simulink model "extend_kalman"  (R2023b)
settings: Solver=FixedStepDiscrete  StartTime=0.0  StopTime=10000  RelTol=1e-3
undefined symbols (not defined in the file or in its folder): BMS_State_Enum, delta_t, dOCV, eta, M, M0, OCV_values, Q, R, R0, sigmaV, sigmaW, soc_values, taw, vbar
libraries: simulink x1
settings Model: DataDictionary=DD_EKF.sldd  Creator=Alkhouly  LastModifiedBy=user
settings OptimizationCC: DefaultParameterBehavior=Inlined  PassReuseOutputArgsAs=Individual arguments  ZeroExternalMemoryAtStartup=off  ZeroInternalMemoryAtStartup=off  OptimizeBlockOrder=speed  DifferentSizesBufferReuse=on  EfficientTunableParamExpr=on
settings DebuggingCC: ParameterTunabilityLossMsg=error  UnconnectedInputMsg=warning  UnconnectedOutputMsg=warning  UnconnectedLineMsg=warning
settings ModelReferenceCC: EnableRefExpFcnMdlSchedulingChecks=on
settings SFSimCC: MATLABDynamicMemAlloc=off
settings RTWCC: Description=Embedded Coder  SystemTargetFile=ert.tlc  GenCodeOnly=on  TemplateMakefile=ert_default_tmf  GenerateReport=on  Toolchain=Texas Instruments Code Composer Studio (C2000)  GenerateWebview=on  GenerateCodeMetricsReport=on  DLArmComputeVersion=19.05
settings CodeAppCC: ForceParamTrailComments=on  IgnoreCustomStorageClasses=off  MaxIdLength=51  OperatorAnnotations=on  SimulinkDataObjDesc=on  SFDataObjDesc=on  MangleLength=4  InsertBlockDesc=on
settings ERTTargetCC: UtilityFuncGeneration=Shared location  SuppressErrorStatus=on  SupportNonFinite=off  SupportComplex=off  ParenthesesLevel=Maximum  CastingMode=Standards  InlinedParameterPlacement=NonHierarchical  ERTCustomFileTemplate=example_file_process.tlc  PreserveExpressionOrder=on  PreserveIfCondition=on  EnableSignedLeftShifts=off  EnableSignedRightShifts=off

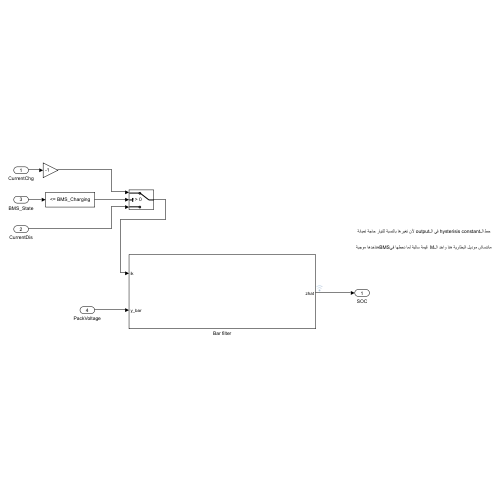
[thumbnail: Simulink's stored preview of the top-level diagram]
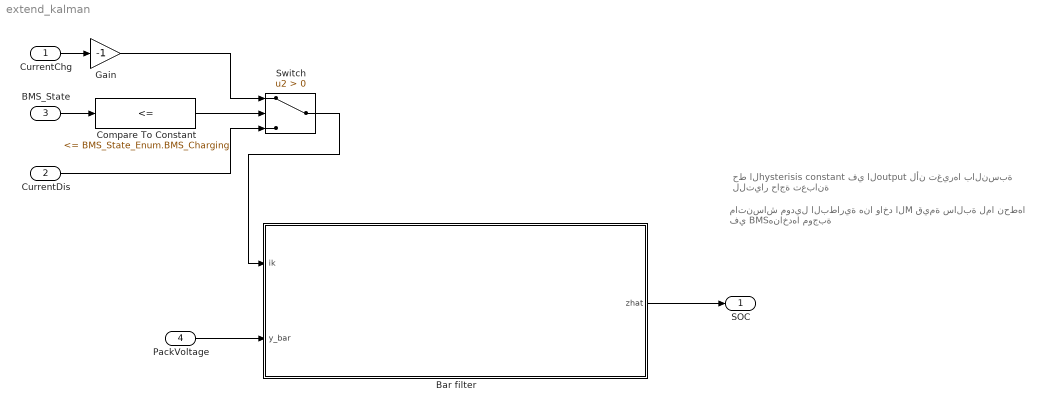
== system extend_kalman ==
  note: ماتنساش موديل البطارية هنا واخد الM قيمة سالبة لما نحطها في BMSهناخدها موجبة
  note: حط الhysterisis constant في الoutput لأن تغيرها بالنسبة للتيار حاجة تعبانة
  CurrentChg : Inport
  CurrentDis : Inport  Port=2
  BMS_State : Inport  Port=3
  PackVoltage : Inport  Port=4
  Bar filter : Subsystem
  Compare To Constant : simulink/Logic and Bit Operations/Compare To Constant  relop=<=  const=BMS_State_Enum.BMS_Charging  OutDataTypeStr=boolean
  Gain : Gain  Gain=-1
  Switch : Switch  Criteria=u2 > Threshold  SaturateOnIntegerOverflow=off  InputSameDT=off
  SOC : Outport
  wires:
  Bar filter/1(zhat) -> SOC/1
  PackVoltage/1 -> Bar filter/2(y_bar)
  CurrentChg/1 -> Gain/1
  CurrentDis/1 -> Switch/3
  Compare To Constant/1 -> Switch/2
  Gain/1 -> Switch/1
  BMS_State/1 -> Compare To Constant/1
  Switch/1 -> Bar filter/1(ik)

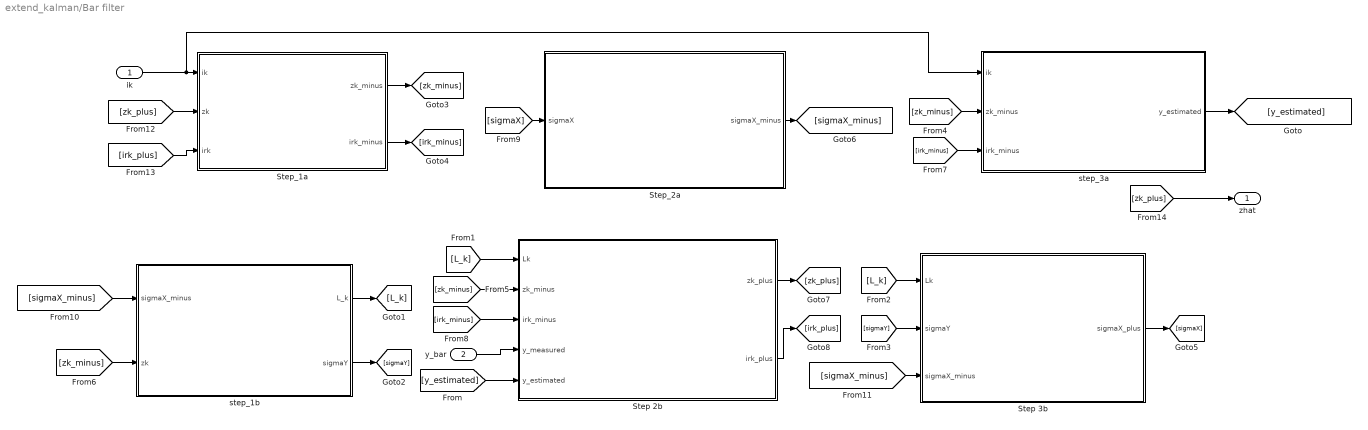
== system extend_kalman/Bar filter ==
  ik : Inport
  y_bar : Inport  Port=2
  Step 2b : Subsystem
  Step 3b : Subsystem
  Step_1a : Subsystem
  Step_2a : Subsystem
  step_1b : Subsystem
  step_3a : Subsystem
  zhat : Outport
  wires:
  ik/1 -> step_3a/1(ik), Step_1a/1(ik)
  y_bar/1 -> Step 2b/4(y_measured)
  step_3a/1(y_estimated) -> [y_estimated]
  [y_estimated] -> Step 2b/5(y_estimated)
  step_1b/1(L_k) -> [L_k]
  [L_k] -> Step 2b/1(Lk)
  [L_k] -> Step 3b/1(Lk)
  step_1b/2(sigmaY) -> [sigmaY]
  [sigmaY] -> Step 3b/2(sigmaY)
  Step_1a/1(zk_minus) -> [zk_minus]
  [zk_minus] -> step_3a/2(zk_minus)
  [zk_minus] -> Step 2b/2(zk_minus)
  [zk_minus] -> step_1b/2(zk)
  Step_1a/2(irk_minus) -> [irk_minus]
  [irk_minus] -> step_3a/3(irk_minus)
  [irk_minus] -> Step 2b/3(irk_minus)
  Step 3b/1(sigmaX_plus) -> [sigmaX]
  [sigmaX] -> Step_2a/1(sigmaX)
  Step_2a/1(sigmaX_minus) -> [sigmaX_minus]
  [sigmaX_minus] -> step_1b/1(sigmaX_minus)
  [sigmaX_minus] -> Step 3b/3(sigmaX_minus)
  Step 2b/1(zk_plus) -> [zk_plus]
  [zk_plus] -> Step_1a/2(zk)
  Step 2b/2(irk_plus) -> [irk_plus]
  [irk_plus] -> Step_1a/3(irk)
  [zk_plus] -> zhat/1

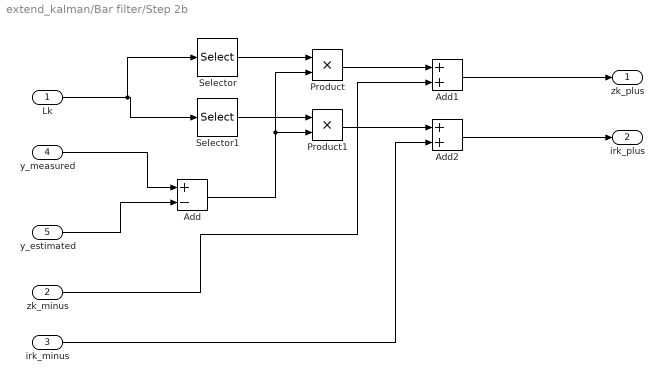
== system extend_kalman/Bar filter/Step 2b ==
  Lk : Inport
  zk_minus : Inport  Port=2
  irk_minus : Inport  Port=3
  y_measured : Inport  Port=4
  y_estimated : Inport  Port=5
  Add : Sum  Inputs=+-
  Add1 : Sum
  Add2 : Sum
  Product : Product
  Product1 : Product
  Selector : Selector  InputPortWidth=2  IndexOptions=Index vector (dialog)  Indices=1  OutputSizes=1
  Selector1 : Selector  InputPortWidth=2  IndexOptions=Index vector (dialog)  Indices=2  OutputSizes=1
  zk_plus : Outport
  irk_plus : Outport  Port=2
  wires:
  y_measured/1 -> Add/1
  y_estimated/1 -> Add/2
  Add/1 -> Product1/2, Product/2
  zk_minus/1 -> Add1/2
  Add1/1 -> zk_plus/1
  Lk/1 -> Selector/1, Selector1/1
  Selector1/1 -> Product1/1
  Selector/1 -> Product/1
  Product/1 -> Add1/1
  Product1/1 -> Add2/1
  irk_minus/1 -> Add2/2
  Add2/1 -> irk_plus/1

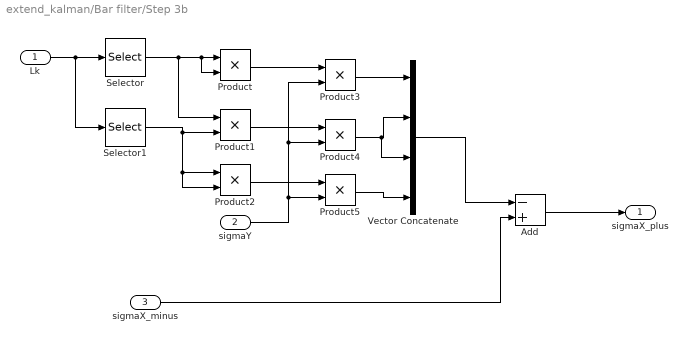
== system extend_kalman/Bar filter/Step 3b ==
  Lk : Inport
  sigmaY : Inport  Port=2
  sigmaX_minus : Inport  Port=3
  Add : Sum  Inputs=-+
  Product{,1..5} (6 alike) : Product
  Selector : Selector  InputPortWidth=2  IndexOptions=Index vector (dialog)  Indices=1  OutputSizes=1
  Selector1 : Selector  InputPortWidth=2  IndexOptions=Index vector (dialog)  Indices=2  OutputSizes=1
  Vector Concatenate : Concatenate  NumInputs=4
  sigmaX_plus : Outport
  wires:
  Vector Concatenate/1 -> Add/1
  sigmaX_minus/1 -> Add/2
  Add/1 -> sigmaX_plus/1
  Lk/1 -> Selector1/1, Selector/1
  Selector/1 -> Product1/1, Product/2, Product/1
  Selector1/1 -> Product1/2, Product2/1, Product2/2
  sigmaY/1 -> Product5/2, Product4/2, Product3/2
  Product/1 -> Product3/1
  Product1/1 -> Product4/1
  Product2/1 -> Product5/1
  Product3/1 -> Vector Concatenate/1
  Product4/1 -> Vector Concatenate/3, Vector Concatenate/2
  Product5/1 -> Vector Concatenate/4

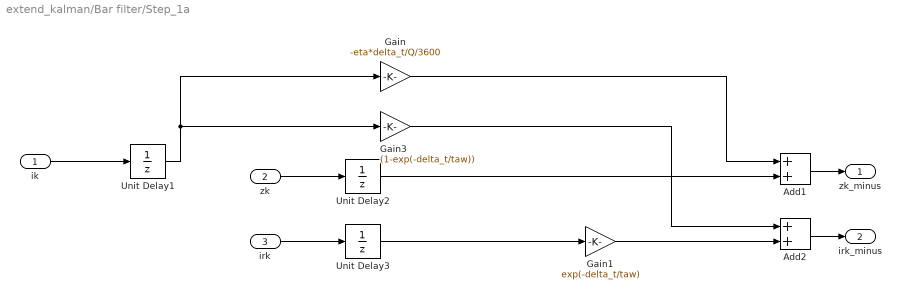
== system extend_kalman/Bar filter/Step_1a ==
  ik : Inport
  zk : Inport  Port=2
  irk : Inport  Port=3
  Add1 : Sum
  Add2 : Sum
  Gain : Gain  Gain=-eta*delta_t/Q/3600
  Gain1 : Gain  Gain=exp(-delta_t/taw)
  Gain3 : Gain  Gain=(1-exp(-delta_t/taw))
  Unit Delay1 : UnitDelay  SampleTime=0.1  HasFrameUpgradeWarning=on
  Unit Delay2 : UnitDelay  InitialCondition=0.5  SampleTime=0.1  HasFrameUpgradeWarning=on
  Unit Delay3 : UnitDelay  SampleTime=0.1  HasFrameUpgradeWarning=on
  zk_minus : Outport
  irk_minus : Outport  Port=2
  wires:
  ik/1 -> Unit Delay1/1
  Unit Delay1/1 -> Gain/1, Gain3/1
  Gain1/1 -> Add2/2
  irk/1 -> Unit Delay3/1
  zk/1 -> Unit Delay2/1
  Gain/1 -> Add1/1
  Gain3/1 -> Add2/1
  Add1/1 -> zk_minus/1
  Add2/1 -> irk_minus/1
  Unit Delay2/1 -> Add1/2
  Unit Delay3/1 -> Gain1/1

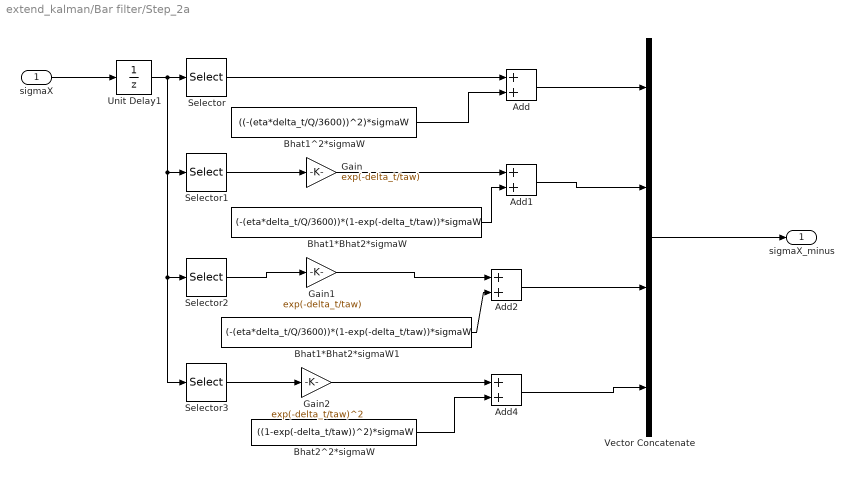
== system extend_kalman/Bar filter/Step_2a ==
  sigmaX : Inport
  Add{,1..2,4} (4 alike) : Sum
  Bhat1*Bhat2*sigmaW : Constant  Value=(-(eta*delta_t/Q/3600))*(1-exp(-delta_t/taw))*sigmaW
  Bhat1*Bhat2*sigmaW1 : Constant  Value=(-(eta*delta_t/Q/3600))*(1-exp(-delta_t/taw))*sigmaW
  Bhat1^2*sigmaW : Constant  Value=((-(eta*delta_t/Q/3600))^2)*sigmaW
  Bhat2^2*sigmaW : Constant  Value=((1-exp(-delta_t/taw))^2)*sigmaW
  Gain : Gain  Gain=exp(-delta_t/taw)
  Gain1 : Gain  Gain=exp(-delta_t/taw)
  Gain2 : Gain  Gain=exp(-delta_t/taw)^2
  Selector : Selector  InputPortWidth=4  IndexOptions=Index vector (dialog)  Indices=1  OutputSizes=1
  Selector1 : Selector  InputPortWidth=4  IndexOptions=Index vector (dialog)  Indices=2  OutputSizes=1
  Selector2 : Selector  InputPortWidth=4  IndexOptions=Index vector (dialog)  Indices=3  OutputSizes=1
  Selector3 : Selector  InputPortWidth=4  IndexOptions=Index vector (dialog)  Indices=4  OutputSizes=1
  Unit Delay1 : UnitDelay  InitialCondition=[0;0;0;0]  SampleTime=0.1  HasFrameUpgradeWarning=on
  Vector Concatenate : Concatenate  NumInputs=4
  sigmaX_minus : Outport
  wires:
  sigmaX/1 -> Unit Delay1/1
  Vector Concatenate/1 -> sigmaX_minus/1
  Unit Delay1/1 -> Selector3/1, Selector2/1, Selector1/1, Selector/1
  Bhat1^2*sigmaW/1 -> Add/2
  Selector/1 -> Add/1
  Selector1/1 -> Gain/1
  Gain/1 -> Add1/1
  Bhat1*Bhat2*sigmaW/1 -> Add1/2
  Selector2/1 -> Gain1/1
  Gain1/1 -> Add2/1
  Bhat1*Bhat2*sigmaW1/1 -> Add2/2
  Selector3/1 -> Gain2/1
  Gain2/1 -> Add4/1
  Bhat2^2*sigmaW/1 -> Add4/2
  Add/1 -> Vector Concatenate/1
  Add1/1 -> Vector Concatenate/2
  Add2/1 -> Vector Concatenate/3
  Add4/1 -> Vector Concatenate/4

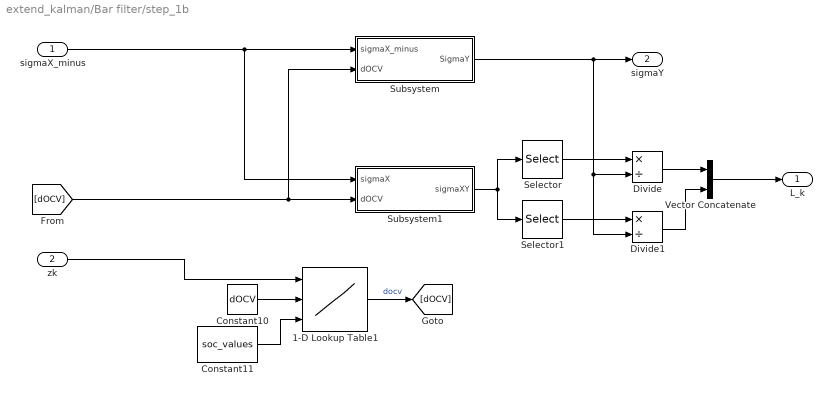
== system extend_kalman/Bar filter/step_1b ==
  sigmaX_minus : Inport
  zk : Inport  Port=2
  1-D Lookup Table1 : Lookup_n-D  NumberOfTableDimensions=1  BreakpointsForDimension1Source=Input port  BreakpointsForDimension1=[-5:5]  TableSource=Input port  Table=tanh([-5:5])  InternalRulePriority=Speed  RndMeth=Simplest
      settings: InputPortMap=u0,p221,p5
  Constant10 : Constant  Value=dOCV
  Constant11 : Constant  Value=soc_values
  Divide : Product  Inputs=*/
  Divide1 : Product  Inputs=*/
  Selector : Selector  InputPortWidth=2  IndexOptions=Index vector (dialog)  Indices=1  OutputSizes=1
  Selector1 : Selector  InputPortWidth=2  IndexOptions=Index vector (dialog)  Indices=2  OutputSizes=1
  Subsystem : Subsystem
  Subsystem1 : Subsystem
  Vector Concatenate : Concatenate
  L_k : Outport
  sigmaY : Outport  Port=2
  wires:
  sigmaX_minus/1 -> Subsystem1/1(sigmaX), Subsystem/1(sigmaX_minus)
  Subsystem/1(SigmaY) -> Divide1/2, Divide/2, sigmaY/1
  zk/1 -> 1-D Lookup Table1/1
  Constant10/1 -> 1-D Lookup Table1/2
  Constant11/1 -> 1-D Lookup Table1/3
  1-D Lookup Table1/1 -> [dOCV]  "docv"
  [dOCV] -> Subsystem/2(dOCV), Subsystem1/2(dOCV)
  Subsystem1/1(sigmaXY) -> Selector1/1, Selector/1
  Selector/1 -> Divide/1
  Selector1/1 -> Divide1/1
  Divide/1 -> Vector Concatenate/1
  Divide1/1 -> Vector Concatenate/2
  Vector Concatenate/1 -> L_k/1

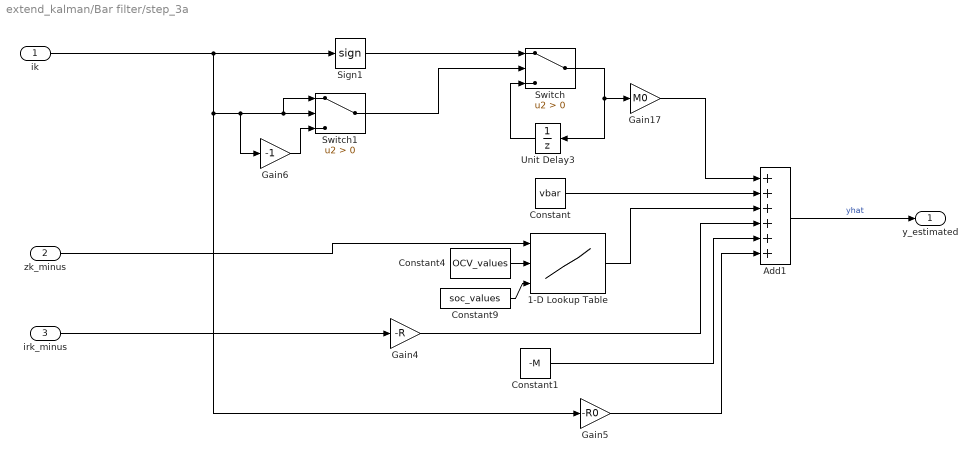
== system extend_kalman/Bar filter/step_3a ==
  ik : Inport
  zk_minus : Inport  Port=2
  irk_minus : Inport  Port=3
  1-D Lookup Table : Lookup_n-D  NumberOfTableDimensions=1  BreakpointsForDimension1Source=Input port  BreakpointsForDimension1=[-5:5]  TableSource=Input port  Table=tanh([-5:5])  InternalRulePriority=Speed  RndMeth=Simplest
      settings: InputPortMap=u0,p221,p5
  Add1 : Sum  Inputs=++++++
  Constant : Constant  Value=vbar
  Constant1 : Constant  Value=-M
  Constant4 : Constant  Value=OCV_values
  Constant9 : Constant  Value=soc_values
  Gain17 : Gain  Gain=M0
  Gain4 : Gain  Gain=-R
  Gain5 : Gain  Gain=-R0
  Gain6 : Gain  Gain=-1
  Sign1 : Signum
  Switch : Switch  Criteria=u2 > Threshold  SaturateOnIntegerOverflow=off  InputSameDT=off
  Switch1 : Switch  Criteria=u2 > Threshold  SaturateOnIntegerOverflow=off  InputSameDT=off
  Unit Delay3 : UnitDelay  SampleTime=-1  HasFrameUpgradeWarning=on
  y_estimated : Outport
  wires:
  Constant9/1 -> 1-D Lookup Table/3
  Add1/1 -> y_estimated/1  "yhat"
  Constant4/1 -> 1-D Lookup Table/2
  Switch1/1 -> Switch/2
  Gain4/1 -> Add1/4
  Sign1/1 -> Switch/1
  Unit Delay3/1 -> Switch/3
  Gain17/1 -> Add1/1
  1-D Lookup Table/1 -> Add1/3
  Constant/1 -> Add1/2
  Switch/1 -> Gain17/1, Unit Delay3/1
  Gain5/1 -> Add1/6
  ik/1 -> Gain5/1, Gain6/1, Switch1/1, Switch1/2, Sign1/1
  Gain6/1 -> Switch1/3
  Constant1/1 -> Add1/5
  zk_minus/1 -> 1-D Lookup Table/1
  irk_minus/1 -> Gain4/1

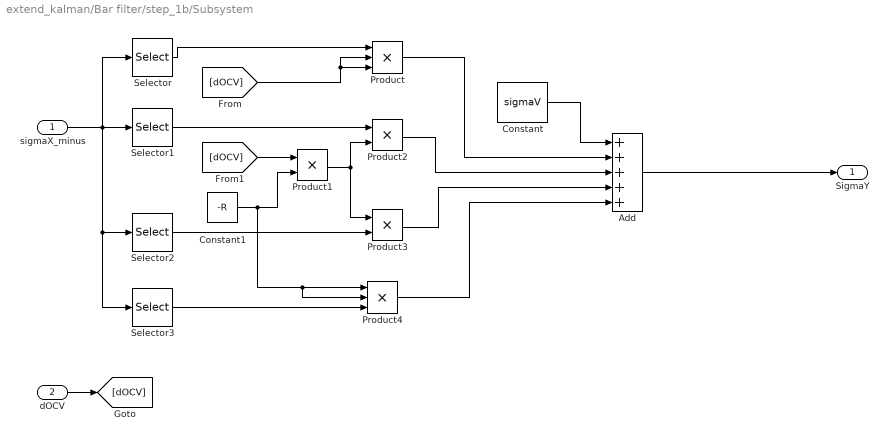
== system extend_kalman/Bar filter/step_1b/Subsystem ==
  sigmaX_minus : Inport
  dOCV : Inport  Port=2
  Add : Sum  Inputs=+++++
  Constant : Constant  Value=sigmaV
  Constant1 : Constant  Value=-R
  Product : Product  Inputs=3
  Product1 : Product
  Product2 : Product
  Product3 : Product
  Product4 : Product  Inputs=3
  Selector : Selector  InputPortWidth=4  IndexOptions=Index vector (dialog)  Indices=1  OutputSizes=1
  Selector1 : Selector  InputPortWidth=4  IndexOptions=Index vector (dialog)  Indices=2  OutputSizes=1
  Selector2 : Selector  InputPortWidth=4  IndexOptions=Index vector (dialog)  Indices=3  OutputSizes=1
  Selector3 : Selector  InputPortWidth=4  IndexOptions=Index vector (dialog)  Indices=4  OutputSizes=1
  SigmaY : Outport
  wires:
  Constant1/1 -> Product4/1, Product4/2, Product1/2
  sigmaX_minus/1 -> Selector3/1, Selector2/1, Selector1/1, Selector/1
  Selector/1 -> Product/1
  [dOCV] -> Product/3, Product/2
  Selector2/1 -> Product3/2
  Selector1/1 -> Product2/1
  Product1/1 -> Product3/1, Product2/2
  Product/1 -> Add/2
  Constant/1 -> Add/1
  Product4/1 -> Add/5
  Product2/1 -> Add/3
  Selector3/1 -> Product4/3
  Product3/1 -> Add/4
  [dOCV] -> Product1/1
  Add/1 -> SigmaY/1
  dOCV/1 -> [dOCV]

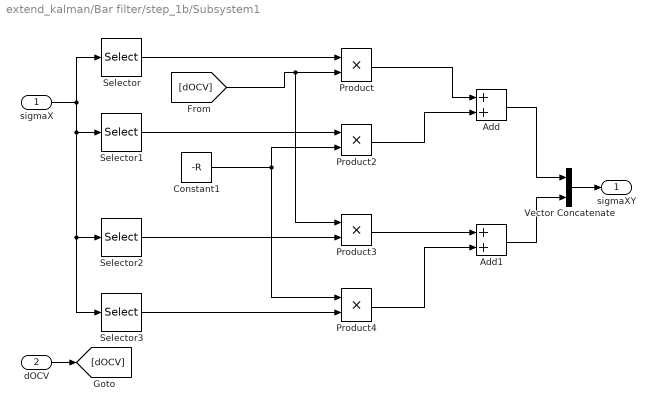
== system extend_kalman/Bar filter/step_1b/Subsystem1 ==
  sigmaX : Inport
  dOCV : Inport  Port=2
  Add : Sum
  Add1 : Sum
  Constant1 : Constant  Value=-R
  Product{,2..4} (4 alike) : Product
  Selector : Selector  InputPortWidth=4  IndexOptions=Index vector (dialog)  Indices=1  OutputSizes=1
  Selector1 : Selector  InputPortWidth=4  IndexOptions=Index vector (dialog)  Indices=2  OutputSizes=1
  Selector2 : Selector  InputPortWidth=4  IndexOptions=Index vector (dialog)  Indices=3  OutputSizes=1
  Selector3 : Selector  InputPortWidth=4  IndexOptions=Index vector (dialog)  Indices=4  OutputSizes=1
  Vector Concatenate : Concatenate
  sigmaXY : Outport
  wires:
  Selector3/1 -> Product4/2
  Product2/1 -> Add/2
  Product4/1 -> Add1/2
  Product3/1 -> Add1/1
  Selector2/1 -> Product3/2
  Selector/1 -> Product/1
  Selector1/1 -> Product2/1
  Product/1 -> Add/1
  dOCV/1 -> [dOCV]
  sigmaX/1 -> Selector/1, Selector3/1, Selector2/1, Selector1/1
  [dOCV] -> Product3/1, Product/2
  Constant1/1 -> Product4/1, Product2/2
  Add/1 -> Vector Concatenate/1
  Add1/1 -> Vector Concatenate/2
  Vector Concatenate/1 -> sigmaXY/1
